simulink subsystem "Direct_Yaw_Command"  (R2023a)
settings: Solver=VariableStepAuto  StartTime=0.0  StopTime=10.0  RelTol=1e-3
undefined symbols (not defined in the file or in its folder): flight_mode
libraries: simulink x1, eeGeneralControl x1
settings Model: Creator=thesa  LastModifiedBy=thesa

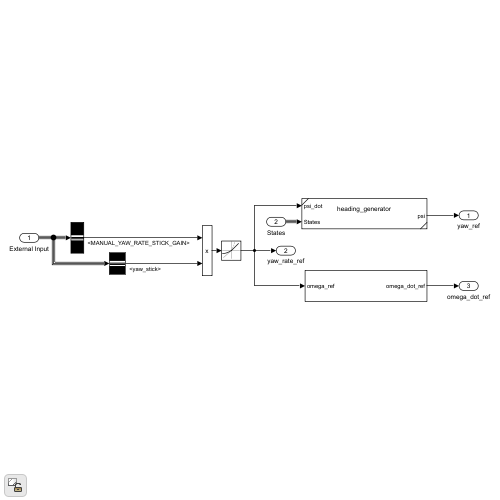
[thumbnail: Simulink's stored preview of the top-level diagram]
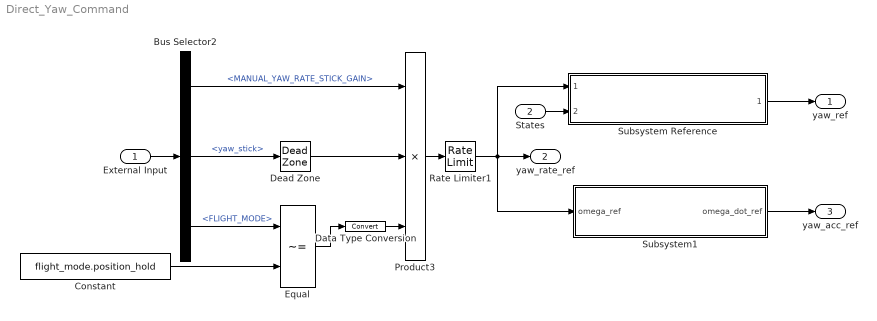
== system Direct_Yaw_Command ==
  External Input : Inport
  States : Inport  Port=2
  Bus Selector2 : BusSelector  OutputSignals=Pilot Input.Parameters.MANUAL_YAW_RATE_STICK_GAIN,Pilot Input.Sticks.yaw_stick,Pilot Input.FLIGHT_MODE
  Constant : Constant  Value=flight_mode.position_hold
  Data Type Conversion : DataTypeConversion  SaturateOnIntegerOverflow=off  RndMeth=Floor
  Dead Zone : DeadZone  LowerValue=-0.05  UpperValue=0.05
  Equal : RelationalOperator  Operator=~=  OutDataTypeStr=boolean  RndMeth=Simplest  InputSameDT=off
  Product3 : Product  Inputs=3
  Rate Limiter1 : RateLimiter  RisingSlewLimit=60*pi/180  FallingSlewLimit=-60*pi/180  SampleTimeMode=inherited
  Subsystem Reference : Subsystem  ReferencedSubsystem=heading_generator
  Subsystem1 : Subsystem
  yaw_ref : Outport
  yaw_rate_ref : Outport  Port=2
  yaw_acc_ref : Outport  Port=3
  wires:
  Subsystem Reference/1 -> yaw_ref/1
  States/1 -> Subsystem Reference/2
  Bus Selector2/2 -> Dead Zone/1  "<yaw_stick>"
  External Input/1 -> Bus Selector2/1
  Rate Limiter1/1 -> yaw_rate_ref/1, Subsystem1/1(omega_ref), Subsystem Reference/1
  Bus Selector2/1 -> Product3/1  "<MANUAL_YAW_RATE_STICK_GAIN>"
  Product3/1 -> Rate Limiter1/1
  Subsystem1/1(omega_dot_ref) -> yaw_acc_ref/1
  Data Type Conversion/1 -> Product3/3
  Equal/1 -> Data Type Conversion/1
  Constant/1 -> Equal/2
  Bus Selector2/3 -> Equal/1  "<FLIGHT_MODE>"
  Dead Zone/1 -> Product3/2

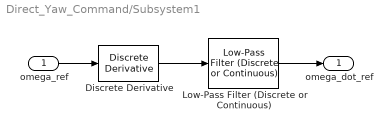
== system Direct_Yaw_Command/Subsystem1 ==
  omega_ref : Inport
  Discrete Derivative : simulink/Discrete/Discrete Derivative  gainval=1.0  ICPrevScaledInput=0.0  OutMin=[]  OutMax=[]  OutDataType=fixdt(1, 16)  OutScaling=2^-10  DoSatur=off
  Low-Pass Filter (Discrete or Continuous) : eeGeneralControl/Low-Pass Filter (Discrete or Continuous)  K=1  T=1/15  B=inf  A=-inf  init_option=Inherited from block input  x0=0  Ts=-1
  omega_dot_ref : Outport
  wires:
  Low-Pass Filter (Discrete or Continuous)/1 -> omega_dot_ref/1
  omega_ref/1 -> Discrete Derivative/1
  Discrete Derivative/1 -> Low-Pass Filter (Discrete or Continuous)/1
